simulink model "SimTF"  (R2023b)
settings: Solver=ode23t  StartTime=0.0  StopTime=SimTime  RelTol=1e-3
values from neighbouring files (symbols this model uses):
  C1 = 1e-3    (= 0.001)    [Sim_SimTF.m]
  C2 = 1e-3    (= 0.001)    [Sim_SimTF.m]
  L1 = 1e-3    (= 0.001)    [Sim_SimTF.m]
  L2 = 2e-3    (= 0.002)    [Sim_SimTF.m]
  R = 0.1    [Sim_SimTF.m]
  SampleTime = 1e-6    (= 1e-06)    [Sim_SimTF.m]
  SimTime = 1    [Sim_SimTF.m]
undefined symbols (not defined in the file or in its folder): C2_ESL, C2_ESR, L_cable, R_cable
libraries: spsSeriesRLCBranchLib x16, spsGroundLib x2, spsImpedanceMeasurementLib x2, simulink x1, spsControlledVoltageSourceLib x1, spsVoltageMeasurementLib x1, sps_lib x1
settings Model: Creator=snow_  LastModifiedBy=snow_
settings DataIOCC: SaveOutput=off  SignalLogging=off  DSMLogging=off  SaveTime=off  ReturnWorkspaceOutputs=off

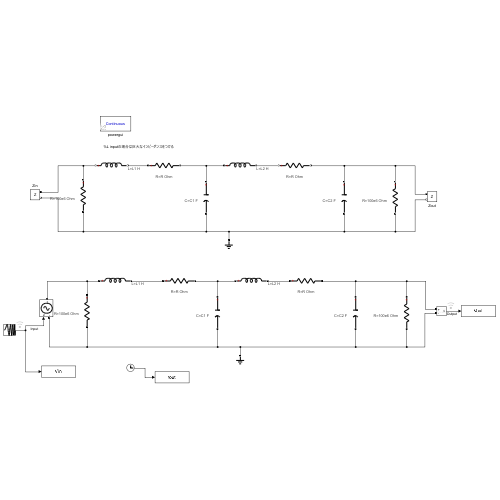
[thumbnail: Simulink's stored preview of the top-level diagram]
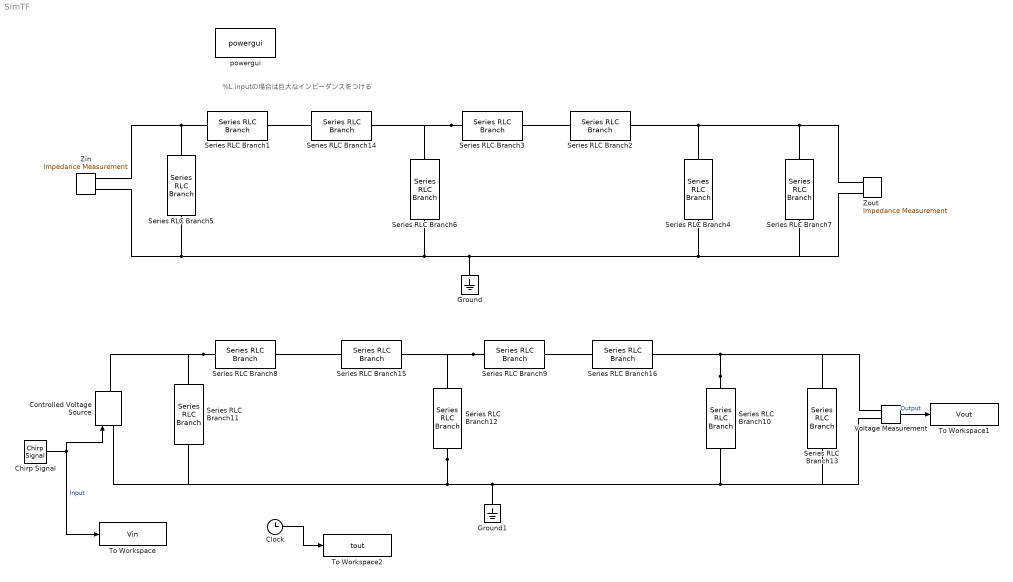
== system SimTF ==
  note: %L inputの場合は巨大なインピーダンスをつける
  Chirp Signal : simulink/Sources/Chirp Signal  f1=10  T=SimTime  f2=10^4
  Clock : Clock
  Controlled Voltage Source : spsControlledVoltageSourceLib/Controlled Voltage Source  Initialize=on  Source_Type=AC  Amplitude=0  Phase=0  Frequency=0  Measurements=None
  Ground : spsGroundLib/Ground  LConnTagsString=a
  Ground1 : spsGroundLib/Ground  LConnTagsString=a
  Series RLC Branch1 : spsSeriesRLCBranchLib/Series RLC Branch  LConnTagsString=__new0  RConnTagsString=__new0  BranchType=L  Resistance=R_cable  Inductance=L1  SetiL0=off  InitialCurrent=0  Capacitance=1e-6  Setx0=off  InitialVoltage=0  Measurements=None
      settings: AttributesFormatString=L=%<Inductance> H
  Series RLC Branch10 : spsSeriesRLCBranchLib/Series RLC Branch  LConnTagsString=__new0  RConnTagsString=__new0  BranchType=C  Resistance=C2_ESR  Inductance=C2_ESL  SetiL0=off  InitialCurrent=0  Capacitance=C2  Setx0=off  InitialVoltage=0  Measurements=None
      settings: AttributesFormatString=C=%<Capacitance> F
  Series RLC Branch{5,7,11,13} (4 alike) : spsSeriesRLCBranchLib/Series RLC Branch  LConnTagsString=__new0  RConnTagsString=__new0  BranchType=R  Resistance=100e6  Inductance=L_cable  SetiL0=off  InitialCurrent=0  Capacitance=1e-6  Setx0=off  InitialVoltage=0  Measurements=None
      settings: AttributesFormatString=R=%<Resistance> Ohm
  Series RLC Branch12 : spsSeriesRLCBranchLib/Series RLC Branch  LConnTagsString=__new0  RConnTagsString=__new0  BranchType=C  Resistance=C2_ESR  Inductance=C2_ESL  SetiL0=off  InitialCurrent=0  Capacitance=C1  Setx0=off  InitialVoltage=0  Measurements=None
      settings: AttributesFormatString=C=%<Capacitance> F
  Series RLC Branch{2,14..16} (4 alike) : spsSeriesRLCBranchLib/Series RLC Branch  LConnTagsString=__new0  RConnTagsString=__new0  BranchType=R  Resistance=R  Inductance=L_cable  SetiL0=off  InitialCurrent=0  Capacitance=1e-6  Setx0=off  InitialVoltage=0  Measurements=None
      settings: AttributesFormatString=R=%<Resistance> Ohm
  Series RLC Branch3 : spsSeriesRLCBranchLib/Series RLC Branch  LConnTagsString=__new0  RConnTagsString=__new0  BranchType=L  Resistance=R_cable  Inductance=L2  SetiL0=off  InitialCurrent=0  Capacitance=1e-6  Setx0=off  InitialVoltage=0  Measurements=None
      settings: AttributesFormatString=L=%<Inductance> H
  Series RLC Branch4 : spsSeriesRLCBranchLib/Series RLC Branch  LConnTagsString=__new0  RConnTagsString=__new0  BranchType=C  Resistance=C2_ESR  Inductance=C2_ESL  SetiL0=off  InitialCurrent=0  Capacitance=C2  Setx0=off  InitialVoltage=0  Measurements=None
      settings: AttributesFormatString=C=%<Capacitance> F
  Series RLC Branch6 : spsSeriesRLCBranchLib/Series RLC Branch  LConnTagsString=__new0  RConnTagsString=__new0  BranchType=C  Resistance=C2_ESR  Inductance=C2_ESL  SetiL0=off  InitialCurrent=0  Capacitance=C1  Setx0=off  InitialVoltage=0  Measurements=None
      settings: AttributesFormatString=C=%<Capacitance> F
  Series RLC Branch8 : spsSeriesRLCBranchLib/Series RLC Branch  LConnTagsString=__new0  RConnTagsString=__new0  BranchType=L  Resistance=R_cable  Inductance=L1  SetiL0=off  InitialCurrent=0  Capacitance=1e-6  Setx0=off  InitialVoltage=0  Measurements=None
      settings: AttributesFormatString=L=%<Inductance> H
  Series RLC Branch9 : spsSeriesRLCBranchLib/Series RLC Branch  LConnTagsString=__new0  RConnTagsString=__new0  BranchType=L  Resistance=R_cable  Inductance=L2  SetiL0=off  InitialCurrent=0  Capacitance=1e-6  Setx0=off  InitialVoltage=0  Measurements=None
      settings: AttributesFormatString=L=%<Inductance> H
  To Workspace : ToWorkspace  VariableName=Vin  SampleTime=SampleTime
  To Workspace1 : ToWorkspace  VariableName=Vout  SampleTime=SampleTime
  To Workspace2 : ToWorkspace  VariableName=tout  SampleTime=SampleTime
  Voltage Measurement : spsVoltageMeasurementLib/Voltage Measurement  PhasorSimulation=off  OutputType=Complex  PSBequivalent=0
  Zin : spsImpedanceMeasurementLib/Impedance Measurement  LConnTagsString=+|-  Factor=1
      settings: LibrarySourceBlock=sps_lib/Sensors and Measurements/Impedance Measurement
  Zout : spsImpedanceMeasurementLib/Impedance Measurement  LConnTagsString=+|-  Factor=1
      settings: LibrarySourceBlock=sps_lib/Sensors and Measurements/Impedance Measurement
  powergui : sps_lib/powergui  Priority=1  SimulationMode=Continuous  SampleTime=50e-6  frequency=60  Iterations=50  frequencyindice=60  Pbase=100e6  ErrMax=1e-4  UnitsV=kV  UnitsW=MW  buscounter=0  FunctionMessages=off  echomessages=off  EnableUseOfTLC=off  CurrentSourceSwitches=off  DisableSnubberDevices=off  DisableRonSwitches=off  DisableVfSwitches=off  DisplayEquations=off  AutomaticDiscreteSolvers=off  SolverType=Tustin/Backward Euler (TBE)  Interpol=off  ExternalGateDelay=off  methode=off  Ts=100  x0status=blocks  SPID=on  SwTol=0  HookPort=off  NonlinearTolerance=1e-4  nMaxIteration=100  ContinueOnMaxIteration=off  RestoreLinks=warning  ResistiveCurrentMeasurement=off  Frange=[0:2:500]  Ylog=off  Xlog=on  ShowGrid=off  save=off  variable=ZData  structure=0  ZoomFFT=off  StartTime=0.0  cycles=1  DisplayStyle=1  fundamental=60  FreqAxis=off  MaxFrequency=1000  frequencyindicesteady=1  RmsSteady=1  display=off
  wires:
  Chirp Signal/1 -> To Workspace/1, Controlled Voltage Source/1  "Input"
  Voltage Measurement/1 -> To Workspace1/1  "Output"
  Clock/1 -> To Workspace2/1
  connections:
  Zin/LConn1 -- Series RLC Branch5/LConn1 -- Series RLC Branch1/LConn1
  Zin/LConn2 -- Series RLC Branch5/RConn1 -- Series RLC Branch7/RConn1 -- Zout/LConn2 -- Series RLC Branch4/RConn1 -- Ground/LConn1 -- Series RLC Branch6/RConn1
  Series RLC Branch3/LConn1 -- Series RLC Branch14/RConn1 -- Series RLC Branch6/LConn1
  Series RLC Branch12/RConn1 -- Ground1/LConn1 -- Voltage Measurement/LConn2 -- Series RLC Branch13/RConn1 -- Series RLC Branch10/RConn1 -- Controlled Voltage Source/LConn1 -- Series RLC Branch11/RConn1
  Series RLC Branch8/LConn1 -- Controlled Voltage Source/RConn1 -- Series RLC Branch11/LConn1
  Series RLC Branch10/LConn1 -- Series RLC Branch16/RConn1 -- Series RLC Branch13/LConn1 -- Voltage Measurement/LConn1
  Series RLC Branch7/LConn1 -- Zout/LConn1 -- Series RLC Branch2/RConn1 -- Series RLC Branch4/LConn1
  Series RLC Branch9/LConn1 -- Series RLC Branch15/RConn1 -- Series RLC Branch12/LConn1
  Series RLC Branch1/RConn1 -- Series RLC Branch14/LConn1
  Series RLC Branch3/RConn1 -- Series RLC Branch2/LConn1
  Series RLC Branch8/RConn1 -- Series RLC Branch15/LConn1
  Series RLC Branch9/RConn1 -- Series RLC Branch16/LConn1
